simulink model "ver_1"  (R2021a)
settings: Solver=VariableStepAuto  StartTime=0.0  StopTime=inf  RelTol=1e-3
model workspace (MAT data in the model file):
  Logfile_Data_Object = robotics.ros.BagSelection
  Logfile_Data_Object.FilePath = 'D:\Documentos\8tvo_semestre\Robotica_movil\Proyecto\Proyecto_robotica_movil\Rosbags\toma1.bag'
  Logfile_Data_Object.StartTime = 4478.693
  Logfile_Data_Object.EndTime = 4597.588
  Logfile_Data_Object.NumMessages = 13517
  Logfile_Data_Object.AvailableTopics = table
  Logfile_Data_Object.AvailableTopics.data{1} = [3217; 3218; 3541; 3541]
  Logfile_Data_Object.AvailableTopics.data{2} = categorical
  Logfile_Data_Object.AvailableTopics.data{2}.categoryNames = {'nav_msgs/Odometry'; 'sensor_msgs/Image'}
  Logfile_Data_Object.AvailableTopics.data{2}.codes = [2; 2; 1; 1]
  Logfile_Data_Object.AvailableTopics.data{3}{1} = '  uint32 Seq
    |   Time Stamp
    |   char FrameId
    | uint32 Height
    | uint32 Width
    | char Encoding
    | uint8 IsBigendian
    | uint32 Step
    | uint8[] Data
    | '
  Logfile_Data_Object.AvailableTopics.data{3}{2} = '  uint32 Seq
    |   Time Stamp
    |   char FrameId
    | uint32 Height
    | uint32 Width
    | char Encoding
    | uint8 IsBigendian
    | uint32 Step
    | uint8[] Data
    | '
  Logfile_Data_Object.AvailableTopics.data{3}{3} = '  uint32 Seq
    |   Time Stamp
    |   char FrameId
    | char ChildFrameId
    | geometry_msgs/PoseWithCovariance Pose
    |   geometry_msgs/Pose Pose
    |     geometry_msgs/Point Position
    |       double X
    |       double Y
    |       double Z
    |     geometry_msgs/Quaternion Orientation
    |       double X
    |       double Y
    |       double Z
    |       double W
    |   double[36] Covariance
    | geometry_msgs/TwistWithCovariance Twist
    |   geometry_msgs/Twist Twist
    |     geometry_msgs/Vector3 Linear
    |       double X
    |       double Y
    |       double Z
    |     geometry_msgs/Vector3 Angular
    |       double X
    |       double Y
    |       double Z
    |   double[36] Covariance
    | '
  Logfile_Data_Object.AvailableTopics.data{3}{4} = '  uint32 Seq
    |   Time Stamp
    |   char FrameId
    | char ChildFrameId
    | geometry_msgs/PoseWithCovariance Pose
    |   geometry_msgs/Pose Pose
    |     geometry_msgs/Point Position
    |       double X
    |       double Y
    |       double Z
    |     geometry_msgs/Quaternion Orientation
    |       double X
    |       double Y
    |       double Z
    |       double W
    |   double[36] Covariance
    | geometry_msgs/TwistWithCovariance Twist
    |   geometry_msgs/Twist Twist
    |     geometry_msgs/Vector3 Linear
    |       double X
    |       double Y
    |       double Z
    |     geometry_msgs/Vector3 Angular
    |       double X
    |       double Y
    |       double Z
    |   double[36] Covariance
    | '
  Logfile_Data_Object.AvailableTopics.ndims = 2
  Logfile_Data_Object.AvailableTopics.nrows = 4
  Logfile_Data_Object.AvailableTopics.rownames = {'/robot1/camera/depth/image_raw'; '/robot1/camera/rgb/image_raw'; '/robot1/odom'; '/robot2/odom'}
  Logfile_Data_Object.AvailableTopics.nvars = 3
  Logfile_Data_Object.AvailableTopics.varnames = {'NumMessages', 'MessageType', 'MessageDefinition'}
  Logfile_Data_Object.AvailableTopics.props.useVariableNamesOriginal = 0
  Logfile_Data_Object.AvailableTopics.props.useDimensionNamesOriginal = 0
  Logfile_Data_Object.AvailableTopics.props.CustomProps = struct()
  Logfile_Data_Object.AvailableTopics.props.VariableCustomProps = struct()
  Logfile_Data_Object.AvailableTopics.props.versionSavedFrom = 4
  Logfile_Data_Object.AvailableTopics.props.minCompatibleVersion = 1
  Logfile_Data_Object.AvailableTopics.props.incompatibilityMsg = ''
  Logfile_Data_Object.AvailableTopics.props.VersionSavedFrom = 4
  Logfile_Data_Object.AvailableTopics.props.Description = ''
  Logfile_Data_Object.AvailableTopics.props.VariableNamesOriginal = {}
  Logfile_Data_Object.AvailableTopics.props.DimensionNames = {'Row', 'Variables'}
  Logfile_Data_Object.AvailableTopics.props.DimensionNamesOriginal = {}
  Logfile_Data_Object.AvailableTopics.props.UserData = []
  Logfile_Data_Object.AvailableTopics.props.VariableDescriptions = {}
  Logfile_Data_Object.AvailableTopics.props.VariableUnits = {}
  Logfile_Data_Object.AvailableTopics.props.VariableContinuity = {}
  Logfile_Data_Object.MessageList = table
  Logfile_Data_Object.MessageList.data{1} = [4478.693 4478.697 4478.727 4478.731 4478.764 4478.764 4478.774 4478.789 4478.793 4478.797 4478.812 4478.823 ... (13517 elements, 13517x1)]
  Logfile_Data_Object.MessageList.data{2} = categorical
  Logfile_Data_Object.MessageList.data{2}.categoryNames = {'/robot1/camera/depth/image_raw'; '/robot1/camera/rgb/image_raw'; '/robot1/odom'; '/robot2/odom'}
  Logfile_Data_Object.MessageList.data{2}.codes = [3 4 3 4 4 3 1 2 3 4 1 2 ... (13517 elements, 13517x1)]
  Logfile_Data_Object.MessageList.data{3} = categorical
  Logfile_Data_Object.MessageList.data{3}.categoryNames = {'sensor_msgs/Image'; 'nav_msgs/Odometry'}
  Logfile_Data_Object.MessageList.data{3}.codes = [2 2 2 2 2 2 1 1 2 2 1 1 ... (13517 elements, 13517x1)]
  Logfile_Data_Object.MessageList.data{4} = [7676 11970 12754 13538 15106 14322 18173 8315272 14536309 14537093 14537877 22832649 ... (13517 elements, 13517x1)]
  Logfile_Data_Object.MessageList.ndims = 2
  Logfile_Data_Object.MessageList.nrows = 13517
  Logfile_Data_Object.MessageList.nvars = 4
  Logfile_Data_Object.MessageList.varnames = {'Time', 'Topic', 'MessageType', 'FileOffset'}
  Logfile_Data_Object.MessageList.props.useVariableNamesOriginal = 0
  Logfile_Data_Object.MessageList.props.useDimensionNamesOriginal = 0
  Logfile_Data_Object.MessageList.props.CustomProps = struct()
  Logfile_Data_Object.MessageList.props.VariableCustomProps = struct()
  Logfile_Data_Object.MessageList.props.versionSavedFrom = 4
  Logfile_Data_Object.MessageList.props.minCompatibleVersion = 1
  Logfile_Data_Object.MessageList.props.incompatibilityMsg = ''
  Logfile_Data_Object.MessageList.props.VersionSavedFrom = 4
  Logfile_Data_Object.MessageList.props.Description = ''
  Logfile_Data_Object.MessageList.props.VariableNamesOriginal = {}
  Logfile_Data_Object.MessageList.props.DimensionNames = {'Row', 'Variables'}
  Logfile_Data_Object.MessageList.props.DimensionNamesOriginal = {}
  Logfile_Data_Object.MessageList.props.UserData = []
  Logfile_Data_Object.MessageList.props.VariableDescriptions = {}
  Logfile_Data_Object.MessageList.props.VariableUnits = {}
  Logfile_Data_Object.MessageList.props.VariableContinuity = {}
  Logfile_Data_Object.TopicTypeMap = containers.Map
  Logfile_Data_Object.TopicTypeMap.serialization.keys = {'/robot1/camera/depth/image_raw', '/robot1/camera/rgb/image_raw', '/robot1/odom', '/robot2/odom'}
  Logfile_Data_Object.TopicTypeMap.serialization.values = {'sensor_msgs/Image', 'sensor_msgs/Image', 'nav_msgs/Odometry', 'nav_msgs/Odometry'}
  Logfile_Data_Object.TopicTypeMap.serialization.uniformity = 1
  Logfile_Data_Object.TopicTypeMap.serialization.keyType = 'char'
  Logfile_Data_Object.TopicTypeMap.serialization.valueType = 'char'
  Logfile_Data_Object.TopicDefinitionMap = containers.Map
  Logfile_Data_Object.TopicDefinitionMap.serialization.keys = {'/robot1/camera/depth/image_raw', '/robot1/camera/rgb/image_raw', '/robot1/odom', '/robot2/odom'}
  Logfile_Data_Object.TopicDefinitionMap.serialization.values{1} = '  uint32 Seq
    |   Time Stamp
    |   char FrameId
    | uint32 Height
    | uint32 Width
    | char Encoding
    | uint8 IsBigendian
    | uint32 Step
    | uint8[] Data
    | '
  Logfile_Data_Object.TopicDefinitionMap.serialization.values{2} = '  uint32 Seq
    |   Time Stamp
    |   char FrameId
    | uint32 Height
    | uint32 Width
    | char Encoding
    | uint8 IsBigendian
    | uint32 Step
    | uint8[] Data
    | '
  Logfile_Data_Object.TopicDefinitionMap.serialization.values{3} = '  uint32 Seq
    |   Time Stamp
    |   char FrameId
    | char ChildFrameId
    | geometry_msgs/PoseWithCovariance Pose
    |   geometry_msgs/Pose Pose
    |     geometry_msgs/Point Position
    |       double X
    |       double Y
    |       double Z
    |     geometry_msgs/Quaternion Orientation
    |       double X
    |       double Y
    |       double Z
    |       double W
    |   double[36] Covariance
    | geometry_msgs/TwistWithCovariance Twist
    |   geometry_msgs/Twist Twist
    |     geometry_msgs/Vector3 Linear
    |       double X
    |       double Y
    |       double Z
    |     geometry_msgs/Vector3 Angular
    |       double X
    |       double Y
    |       double Z
    |   double[36] Covariance
    | '
  Logfile_Data_Object.TopicDefinitionMap.serialization.values{4} = '  uint32 Seq
    |   Time Stamp
    |   char FrameId
    | char ChildFrameId
    | geometry_msgs/PoseWithCovariance Pose
    |   geometry_msgs/Pose Pose
    |     geometry_msgs/Point Position
    |       double X
    |       double Y
    |       double Z
    |     geometry_msgs/Quaternion Orientation
    |       double X
    |       double Y
    |       double Z
    |       double W
    |   double[36] Covariance
    | geometry_msgs/TwistWithCovariance Twist
    |   geometry_msgs/Twist Twist
    |     geometry_msgs/Vector3 Linear
    |       double X
    |       double Y
    |       double Z
    |     geometry_msgs/Vector3 Angular
    |       double X
    |       double Y
    |       double Z
    |   double[36] Covariance
    | '
  Logfile_Data_Object.TopicDefinitionMap.serialization.uniformity = 1
  Logfile_Data_Object.TopicDefinitionMap.serialization.keyType = 'char'
  Logfile_Data_Object.TopicDefinitionMap.serialization.valueType = 'char'
  Logfile_Data_Object.messageTypeMap = containers.Map
  Logfile_Data_Object.messageTypeMap.serialization.keys = {}
  Logfile_Data_Object.messageTypeMap.serialization.values = {}
  Logfile_Data_Object.messageTypeMap.serialization.uniformity = 0
  Logfile_Data_Object.messageTypeMap.serialization.keyType = 'char'
  Logfile_Data_Object.messageTypeMap.serialization.valueType = 'any'
  Logfile_Data_Object.Parser = robotics.ros.internal.tf.TransformationTreeParser
  Logfile_Data_Object.Parser.UseObjectMsg = 1
  Logfile_Path = 'D:\Documentos\8tvo_semestre\Robotica_movil\Proyecto\Proyecto_robotica_movil\Rosbags\toma1.bag'
  Logfile_Playback_Duration = 30
  Logfile_Playback_Offset = 83
  SL_ROS_VariableLengthArrays_MaxSizes.CommonInfo.ArrayTruncateAction = 'EmitWarning'
  SL_ROS_VariableLengthArrays_MaxSizes.MsgTypeMap = containers.Map
  SL_ROS_VariableLengthArrays_MaxSizes.MsgTypeMap.serialization.keys = {'sensor_msgs/Image'}
  SL_ROS_VariableLengthArrays_MaxSizes.MsgTypeMap.serialization.values{1}(1).PropertyName = 'Data'
  SL_ROS_VariableLengthArrays_MaxSizes.MsgTypeMap.serialization.values{1}(1).DataType = 'uint8'
  SL_ROS_VariableLengthArrays_MaxSizes.MsgTypeMap.serialization.values{1}(1).MaxLength = 8294400
  SL_ROS_VariableLengthArrays_MaxSizes.MsgTypeMap.serialization.values{1}(2).PropertyName = 'Encoding'
  SL_ROS_VariableLengthArrays_MaxSizes.MsgTypeMap.serialization.values{1}(2).DataType = 'uint8'
  SL_ROS_VariableLengthArrays_MaxSizes.MsgTypeMap.serialization.values{1}(2).MaxLength = 128
  SL_ROS_VariableLengthArrays_MaxSizes.MsgTypeMap.serialization.uniformity = 0
  SL_ROS_VariableLengthArrays_MaxSizes.MsgTypeMap.serialization.keyType = 'char'
  SL_ROS_VariableLengthArrays_MaxSizes.MsgTypeMap.serialization.valueType = 'any'
libraries: robotlib x6, visiontextngfix x3, visionconversions x2, simulink x2
settings Model: Creator=andres  LastModifiedBy=xboxk

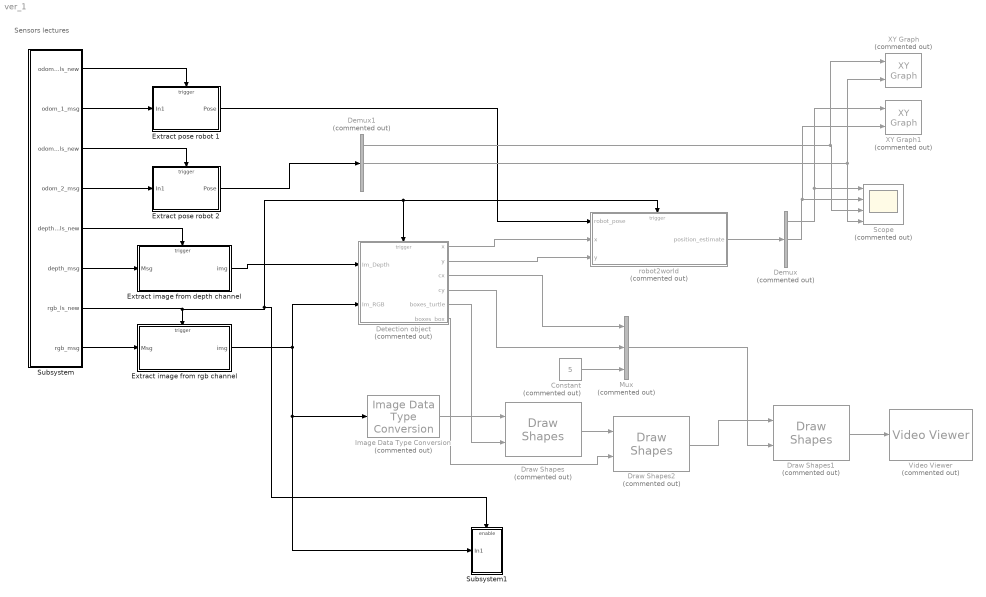
== system ver_1 ==
  note: Sensors lectures
  Constant : Constant  Commented=on  Value=5
  Demux : Demux  Commented=on  Outputs=3
  Demux1 : Demux  Commented=on  Outputs=3
  Detection object : Subsystem  Commented=on
  Draw Shapes : visiontextngfix/Draw Shapes  Commented=on  shape=Rectangles  fill=off  lineWidth=2  fillClrSource=Specify via dialog  display=User-specified value  intensity=200  color=[255 0 0]  opacity=0.6  viewport=Entire image  antialiasing=off  inType=Obsolete  imagePorts=One multidimensional signal  roundingMode=Floor  overflowMode=off  memoryMode=Specify word length  memoryWordLength=16  prodOutputMode=Binary point scaling  prodOutputWordLength=32  prodOutputFracLength=14  memoryFracLength=15
  Draw Shapes1 : visiontextngfix/Draw Shapes  Commented=on  shape=Circles  fill=off  lineWidth=2  fillClrSource=Specify via dialog  display=User-specified value  intensity=200  color=[255 0 0]  opacity=0.6  viewport=Entire image  antialiasing=off  inType=Obsolete  imagePorts=One multidimensional signal  roundingMode=Floor  overflowMode=off  memoryMode=Specify word length  memoryWordLength=16  prodOutputMode=Binary point scaling  prodOutputWordLength=32  prodOutputFracLength=14  memoryFracLength=15
  Draw Shapes2 : visiontextngfix/Draw Shapes  Commented=on  shape=Rectangles  fill=off  lineWidth=2  fillClrSource=Specify via dialog  display=User-specified value  intensity=200  color=[0 0 255]  opacity=0.6  viewport=Entire image  antialiasing=off  inType=Obsolete  imagePorts=One multidimensional signal  roundingMode=Floor  overflowMode=off  memoryMode=Specify word length  memoryWordLength=16  prodOutputMode=Binary point scaling  prodOutputWordLength=32  prodOutputFracLength=14  memoryFracLength=15
  Extract image from depth channel : Subsystem
  Extract image from rgb channel : Subsystem
  Extract pose robot 1 : Subsystem
  Extract pose robot 2 : Subsystem
  Image Data Type Conversion : visionconversions/Image Data Type Conversion  Commented=on  outDT=single  isSigned=on  wordLen=16  numFracBits=0
      settings: SourceProductBaseCode=VP
  Mux : Mux  Commented=on  Inputs=3
  Scope : Scope  Commented=on  NumInputPorts=4
  Subsystem : Subsystem  mask{Sample_time=0.01}
      mask prompts: Sample_time "Sample time"
  Subsystem1 : Subsystem
  Video Viewer : VideoViewer  Commented=on  FigPos=[1 822 1536 724]
  XY Graph : simulink/Sinks/XY Graph  Commented=on  xmin=-10  xmax=10  ymin=-10  ymax=10  st=-1
  XY Graph1 : simulink/Sinks/XY Graph  Commented=on  xmin=-10  xmax=10  ymin=-10  ymax=10  st=-1
  robot2world : Subsystem  Commented=on
  wires:
  Subsystem/2(odom_1_msg) -> Extract pose robot 1/1(In1)
  Subsystem/1(odom_1_ls_new) -> Extract pose robot 1/Trigger
  Subsystem/3(odom_2_ls_new) -> Extract pose robot 2/Trigger
  Subsystem/4(odom_2_msg) -> Extract pose robot 2/1(In1)
  Subsystem/7(rgb_ls_new) -> Subsystem1/Enable, Detection object/Trigger, robot2world/Trigger, Extract image from rgb channel/Trigger
  Subsystem/8(rgb_msg) -> Extract image from rgb channel/1(Msg)
  Subsystem/6(depth_msg) -> Extract image from depth channel/1(Msg)
  Subsystem/5(depth_ls_new) -> Extract image from depth channel/Trigger
  Extract image from depth channel/1(img) -> Detection object/1(Im_Depth)
  Extract image from rgb channel/1(img) -> Detection object/2(Im_RGB), Subsystem1/1(In1), Image Data Type Conversion/1
  Image Data Type Conversion/1 -> Draw Shapes/1
  Detection object/5(boxes_turtle) -> Draw Shapes/2
  Detection object/3(cx) -> Mux/1
  Detection object/4(cy) -> Mux/2
  Constant/1 -> Mux/3
  Mux/1 -> Draw Shapes1/2
  Draw Shapes1/1 -> Video Viewer/1
  Detection object/1(x) -> robot2world/2(x)
  Detection object/2(y) -> robot2world/3(y)
  Extract pose robot 1/1(Pose) -> robot2world/1(robot_pose)
  robot2world/1(position_estimate) -> Demux/1
  Demux/2 -> XY Graph1/2, Scope/2
  Demux/1 -> XY Graph1/1, Scope/1
  Extract pose robot 2/1(Pose) -> Demux1/1
  Demux1/1 -> XY Graph/1, Scope/3
  Demux1/2 -> Scope/4, XY Graph/2
  Draw Shapes/1 -> Draw Shapes2/1
  Draw Shapes2/1 -> Draw Shapes1/1
  Detection object/6(boxes_box) -> Draw Shapes2/2

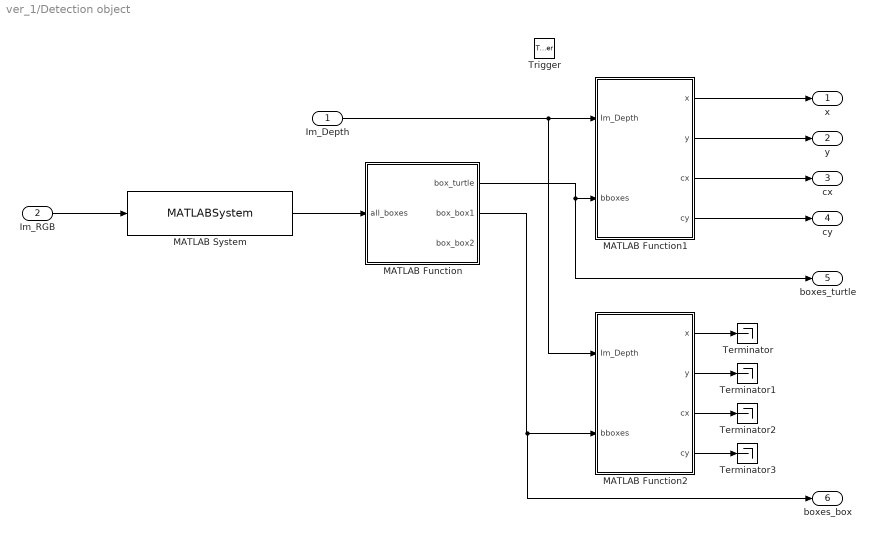
== system ver_1/Detection object ==
  Im_Depth : Inport
  Im_RGB : Inport  Port=2
  Trigger : TriggerPort  VariantControl=(inherit)  PortDimensions=1
  MATLAB Function : MATLAB Function  TreatAsAtomicUnit=on
  MATLAB Function1 : MATLAB Function  TreatAsAtomicUnit=on
  MATLAB Function2 : MATLAB Function  TreatAsAtomicUnit=on
  MATLAB System : MATLABSystem  System=yolov3  yolov=[]  SimulateUsing=Interpreted execution
      mask Type: yolov3
      mask Display:
      | disp('yolov3');
      | port_label('input',1,'Im_RGB');
      | port_label('output',1,'bboxes');
  Terminator{,1..3} (4 alike) : Terminator
  x : Outport
  y : Outport  Port=2
  cx : Outport  Port=3
  cy : Outport  Port=4
  boxes_turtle : Outport  Port=5
  boxes_box : Outport  Port=6
  wires:
  Im_RGB/1 -> MATLAB System/1
  Im_Depth/1 -> MATLAB Function2/1(Im_Depth), MATLAB Function1/1(Im_Depth)
  MATLAB Function1/1(x) -> x/1
  MATLAB Function1/2(y) -> y/1
  MATLAB Function1/3(cx) -> cx/1
  MATLAB Function1/4(cy) -> cy/1
  MATLAB System/1 -> MATLAB Function/1(all_boxes)
  MATLAB Function/1(box_turtle) -> boxes_turtle/1, MATLAB Function1/2(bboxes)
  MATLAB Function/2(box_box1) -> boxes_box/1, MATLAB Function2/2(bboxes)
  MATLAB Function2/1(x) -> Terminator/1
  MATLAB Function2/2(y) -> Terminator1/1
  MATLAB Function2/3(cx) -> Terminator2/1
  MATLAB Function2/4(cy) -> Terminator3/1

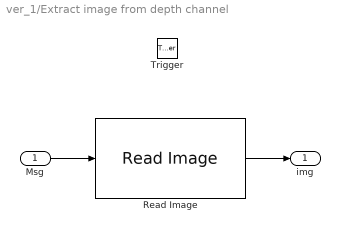
== system ver_1/Extract image from depth channel ==
  Msg : Inport
  Trigger : TriggerPort  VariantControl=(inherit)  PortDimensions=1
  Read Image : robotlib/Read Image  MaximumImageSize=[1080 , 1920]  ImageEncoding=32fc1  ShowAlphaOutput=off  ShowErrorCodeOutput=off  VariableSizeOutputs=off
      settings: SourceProductBaseCode=RR
  img : Outport
  wires:
  Msg/1 -> Read Image/1
  Read Image/1 -> img/1

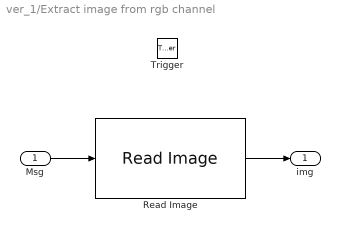
== system ver_1/Extract image from rgb channel ==
  Msg : Inport
  Trigger : TriggerPort  VariantControl=(inherit)  PortDimensions=1
  Read Image : robotlib/Read Image  MaximumImageSize=[1080 , 1920]  ImageEncoding=rgb8  ShowAlphaOutput=off  ShowErrorCodeOutput=off  VariableSizeOutputs=off
      settings: SourceProductBaseCode=RR
  img : Outport
  wires:
  Read Image/1 -> img/1
  Msg/1 -> Read Image/1

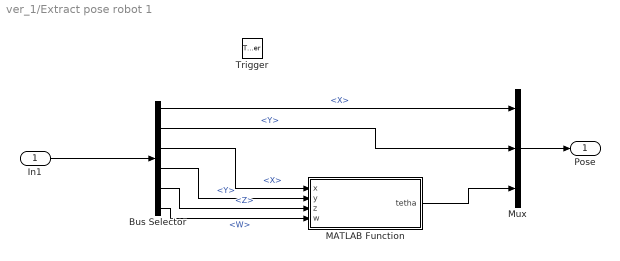
== system ver_1/Extract pose robot 1 ==
  In1 : Inport
  Trigger : TriggerPort  VariantControl=(inherit)  PortDimensions=1
  Bus Selector : BusSelector  OutputSignals=Pose.Pose.Position.X,Pose.Pose.Position.Y,Pose.Pose.Orientation.X,Pose.Pose.Orientation.Y,Pose.Pose.Orientation.Z,Pose.Pose.Orientation.W
  MATLAB Function : MATLAB Function  TreatAsAtomicUnit=on
  Mux : Mux  Inputs=3
  Pose : Outport
  wires:
  MATLAB Function/1(tetha) -> Mux/3
  Bus Selector/2 -> Mux/2  "<Y>"
  In1/1 -> Bus Selector/1
  Bus Selector/3 -> MATLAB Function/1(x)  "<X>"
  Bus Selector/4 -> MATLAB Function/2(y)  "<Y>"
  Bus Selector/5 -> MATLAB Function/3(z)  "<Z>"
  Bus Selector/6 -> MATLAB Function/4(w)  "<W>"
  Bus Selector/1 -> Mux/1  "<X>"
  Mux/1 -> Pose/1

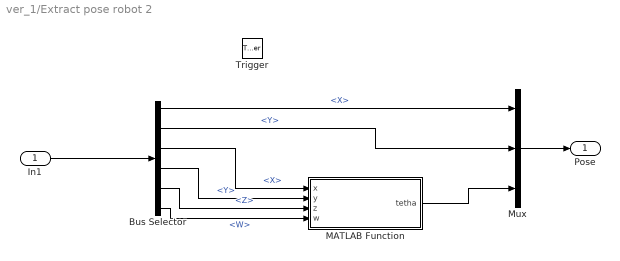
== system ver_1/Extract pose robot 2 ==
  In1 : Inport
  Trigger : TriggerPort  VariantControl=(inherit)  PortDimensions=1
  Bus Selector : BusSelector  OutputSignals=Pose.Pose.Position.X,Pose.Pose.Position.Y,Pose.Pose.Orientation.X,Pose.Pose.Orientation.Y,Pose.Pose.Orientation.Z,Pose.Pose.Orientation.W
  MATLAB Function : MATLAB Function  TreatAsAtomicUnit=on
  Mux : Mux  Inputs=3
  Pose : Outport
  wires:
  Mux/1 -> Pose/1
  Bus Selector/1 -> Mux/1  "<X>"
  Bus Selector/6 -> MATLAB Function/4(w)  "<W>"
  Bus Selector/5 -> MATLAB Function/3(z)  "<Z>"
  Bus Selector/4 -> MATLAB Function/2(y)  "<Y>"
  Bus Selector/3 -> MATLAB Function/1(x)  "<X>"
  In1/1 -> Bus Selector/1
  Bus Selector/2 -> Mux/2  "<Y>"
  MATLAB Function/1(tetha) -> Mux/3

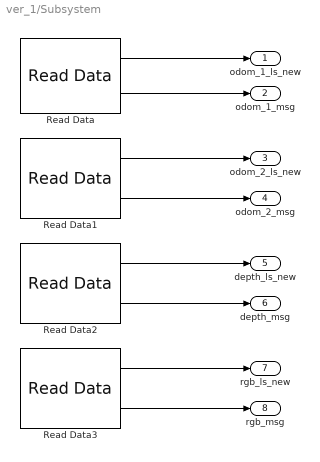
== system ver_1/Subsystem ==
  Read Data : robotlib/Read Data  topic=/robot1/odom  sampleTime=Sample_time  logfileType=rosbag  modelName=ver_1  msgType=nav_msgs/Odometry
      settings: SourceProductBaseCode=RR
  Read Data1 : robotlib/Read Data  topic=/robot2/odom  sampleTime=Sample_time  logfileType=rosbag  modelName=ver_1  msgType=nav_msgs/Odometry
      settings: SourceProductBaseCode=RR
  Read Data2 : robotlib/Read Data  topic=/robot1/camera/depth/image_raw  sampleTime=Sample_time  logfileType=rosbag  modelName=ver_1  msgType=sensor_msgs/Image
      settings: SourceProductBaseCode=RR
  Read Data3 : robotlib/Read Data  topic=/robot1/camera/rgb/image_raw  sampleTime=Sample_time  logfileType=rosbag  modelName=ver_1  msgType=sensor_msgs/Image
      settings: SourceProductBaseCode=RR
  odom_1_ls_new : Outport
  odom_1_msg : Outport  Port=2
  odom_2_ls_new : Outport  Port=3
  odom_2_msg : Outport  Port=4
  depth_ls_new : Outport  Port=5
  depth_msg : Outport  Port=6
  rgb_ls_new : Outport  Port=7
  rgb_msg : Outport  Port=8
  wires:
  Read Data2/1 -> depth_ls_new/1
  Read Data1/1 -> odom_2_ls_new/1
  Read Data/1 -> odom_1_ls_new/1
  Read Data1/2 -> odom_2_msg/1
  Read Data/2 -> odom_1_msg/1
  Read Data2/2 -> depth_msg/1
  Read Data3/1 -> rgb_ls_new/1
  Read Data3/2 -> rgb_msg/1

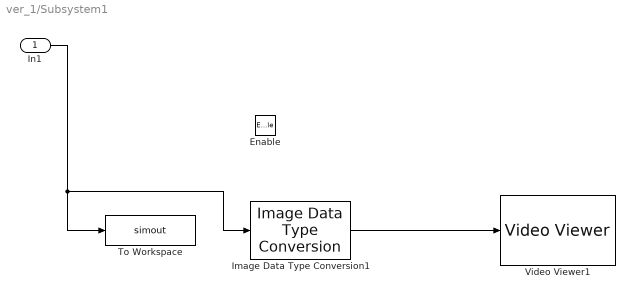
== system ver_1/Subsystem1 ==
  In1 : Inport
  Enable : EnablePort
  Image Data Type Conversion1 : visionconversions/Image Data Type Conversion  outDT=single  isSigned=on  wordLen=16  numFracBits=0
      settings: SourceProductBaseCode=VP
  To Workspace : ToWorkspace  VariableName=simout  SaveFormat=Structure  SampleTime=-1
  Video Viewer1 : VideoViewer  FigPos=[1 822 1536 724]
  wires:
  In1/1 -> Image Data Type Conversion1/1, To Workspace/1
  Image Data Type Conversion1/1 -> Video Viewer1/1

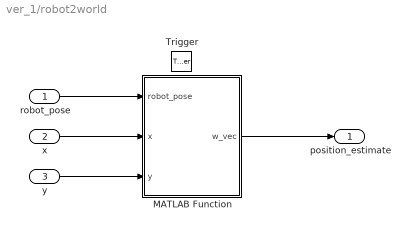
== system ver_1/robot2world ==
  robot_pose : Inport
  x : Inport  Port=2
  y : Inport  Port=3
  Trigger : TriggerPort  VariantControl=(inherit)  PortDimensions=1
  MATLAB Function : MATLAB Function  TreatAsAtomicUnit=on
  position_estimate : Outport
  wires:
  MATLAB Function/1(w_vec) -> position_estimate/1
  robot_pose/1 -> MATLAB Function/1(robot_pose)
  x/1 -> MATLAB Function/2(x)
  y/1 -> MATLAB Function/3(y)

== matlab function ver_1/Extract pose robot 2/MATLAB Function ==
  data: x input double size=1; tetha output double size=1; y input double size=1; z input double size=1; w input double size=1
function tetha = quaternion2angulo(x,y,z,w)
    tetha = atan2(2.0*(w*z + x*y), 1.0 - 2.0*(y^2 + z^2));

== matlab function ver_1/Extract pose robot 1/MATLAB Function ==
  data: x input double size=1; tetha output double size=1; y input double size=1; z input double size=1; w input double size=1
function tetha = quaternion2angulo(x,y,z,w)
    tetha = atan2(2.0*(w*z + x*y), 1.0 - 2.0*(y^2 + z^2));

== matlab function ver_1/robot2world/MATLAB Function ==
  data: robot_pose input double size=3,1; w_vec output double size=3,1; x input double size=1; y input double size=1
function w_vec= fcn(robot_pose,x,y)

w_vec= diferencial_robot.transformar_robot2wordl([robot_pose(1);robot_pose(2);0],robot_pose(3),[x;y;0]);

== matlab function ver_1/Detection object/MATLAB Function1 ==
  data: Im_Depth input single size=1080 ,1920; x output double size=1; bboxes input single size=1,4; y output double size=1; cx output double size=1; cy output double size=1
function [x,y,cx,cy] = fcn(Im_Depth,bboxes)
    
    [x,y,cx,cy]= calculo_depth_simulink(bboxes,Im_Depth);

== matlab function ver_1/Detection object/MATLAB Function ==
  data: all_boxes input single size=3,4; box_turtle output single size=1,4; box_box1 output single size=1,4; box_box2 output single size=1,4
function [box_turtle,box_box1,box_box2]= fcn(all_boxes)

box_turtle = all_boxes(1,:);
box_box1 = all_boxes(2,:);
box_box2 = all_boxes(3,:);

== matlab function ver_1/Detection object/MATLAB Function2 ==
  data: Im_Depth input single size=1080 ,1920; x output double size=1; bboxes input single size=1,4; y output double size=1; cx output double size=1; cy output double size=1
function [x,y,cx,cy] = fcn(Im_Depth,bboxes)
    
    [x,y,cx,cy]= calculo_depth_simulink(bboxes,Im_Depth);
